simulink model "mtr_fuzzy_mdl"  (R2022b)
settings: Solver=VariableStepAuto  StartTime=0.0  StopTime=1.5  RelTol=1e-3
libraries: fuzblock x1
settings Model: Creator=javnson  LastModifiedBy=javnson

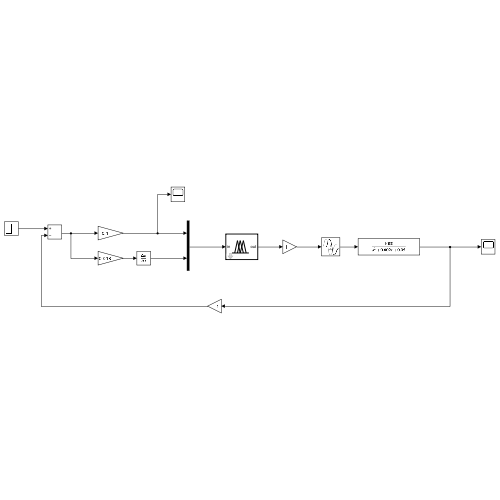
[thumbnail: Simulink's stored preview of the top-level diagram]
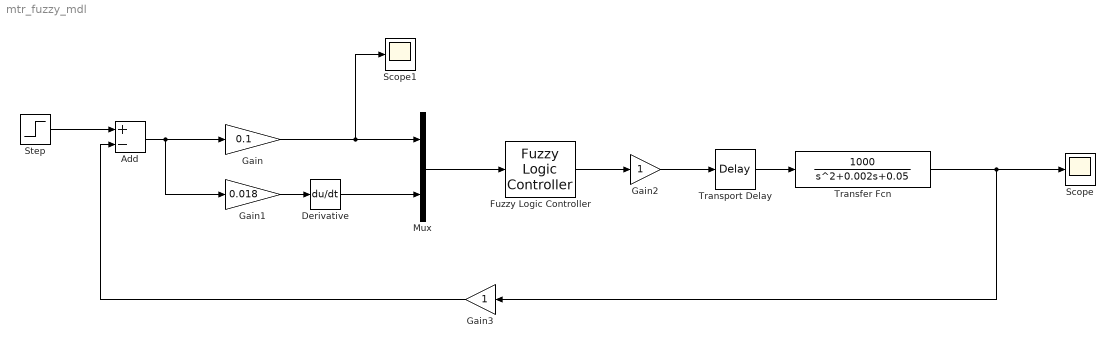
== system mtr_fuzzy_mdl ==
  Add : Sum  Inputs=+-
  Derivative : Derivative
  Fuzzy Logic Controller : fuzblock/Fuzzy Logic  Controller  FIS='mtr_fuzzy_dsn.fis'  OutputSampleNumber=101  DataType=double  FuzzifiedInputs=off  RuleFiringStrengths=off  RuleOutputs=off  AggregatedOutputs=off  SimulateUsing=Interpreted execution  OutOfRangeInputValueMessage=warning  NoRuleFiredMessage=warning  EmptyOutputFuzzySetMessage=warning
  Gain : Gain  Gain=0.1
  Gain1 : Gain  Gain=0.018
  Gain2 : Gain
  Gain3 : Gain
  Mux : Mux  Inputs=2
  Scope : Scope
  Scope1 : Scope
  Step : Step  Time=0.05  SampleTime=0
  Transfer Fcn : TransferFcn  Numerator=[1000]  Denominator=[1 0.002 0.05]
  Transport Delay : TransportDelay  DelayTime=0.05
  wires:
  Step/1 -> Add/1
  Gain1/1 -> Derivative/1
  Add/1 -> Gain/1, Gain1/1
  Derivative/1 -> Mux/2
  Gain/1 -> Scope1/1, Mux/1
  Mux/1 -> Fuzzy Logic Controller/1
  Fuzzy Logic Controller/1 -> Gain2/1
  Gain2/1 -> Transport Delay/1
  Transport Delay/1 -> Transfer Fcn/1
  Transfer Fcn/1 -> Gain3/1, Scope/1
  Gain3/1 -> Add/2
